simulink model "PenduloCarro"  (R2017b)
settings: Solver=ode4  StartTime=0.0  StopTime=10  FixedStep=0.0001  RelTol=1e-3
values from neighbouring files (symbols this model uses):
  g = 9.81    [PenduloInvertido.m]
  l = 0.5    [PenduloInvertido.m]
  m = 0.1    [PenduloInvertido.m]
  M = 2    [PenduloInvertido.m]
settings Model: Creator=Benjamin Nicolas  LastModifiedBy=Benjamin Nicolas

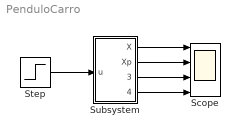
== system PenduloCarro ==
  Scope : Scope  NumInputPorts=4
  Step : Step  Time=0  SampleTime=0
  Subsystem : Subsystem
  wires:
  Subsystem/1(X) -> Scope/1
  Subsystem/2(Xp) -> Scope/2
  Subsystem/3(Theta) -> Scope/3
  Subsystem/4(Thetap) -> Scope/4
  Step/1 -> Subsystem/1("u ")

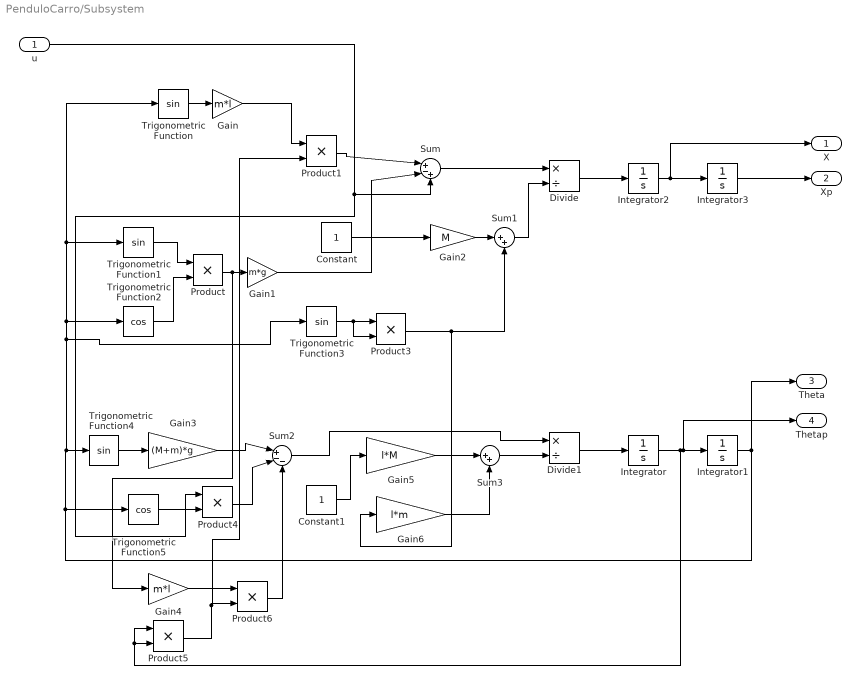
== system PenduloCarro/Subsystem ==
  "u " : Inport
  Constant : Constant
  Constant1 : Constant
  Divide : Product  Inputs=*/
  Divide1 : Product  Inputs=*/
  Gain : Gain  Gain=m*l
  Gain1 : Gain  Gain=m*g
  Gain2 : Gain  Gain=M
  Gain3 : Gain  Gain=(M+m)*g
  Gain4 : Gain  Gain=m*l
  Gain5 : Gain  Gain=l*M
  Gain6 : Gain  Gain=l*m
  Integrator{,1..3} (4 alike) : Integrator
  Product{,1,3..6} (6 alike) : Product
  Sum : Sum  Inputs=|+-+
  Sum1 : Sum  Inputs=|++
  Sum2 : Sum  Inputs=|+--
  Sum3 : Sum  Inputs=|++
  Trigonometric Function{,1,3..4} (4 alike) : Trigonometry
  Trigonometric Function2 : Trigonometry  Operator=cos
  Trigonometric Function5 : Trigonometry  Operator=cos
  X : Outport
  Xp : Outport  Port=2
  Theta : Outport  Port=3
  Thetap : Outport  Port=4
  wires:
  Gain3/1 -> Sum2/1
  Gain4/1 -> Product6/1
  Product3/1 -> Gain6/1, Sum1/2
  Gain1/1 -> Sum/2
  Trigonometric Function3/1 -> Product3/2, Product3/1
  Sum1/1 -> Divide/2
  Gain2/1 -> Sum1/1
  Product5/1 -> Product1/2, Product6/2
  Product6/1 -> Sum2/3
  Sum/1 -> Divide/1
  Product/1 -> Gain4/1, Gain1/1
  Trigonometric Function1/1 -> Product/1
  Gain6/1 -> Sum3/2
  Constant1/1 -> Gain5/1
  Trigonometric Function2/1 -> Product/2
  Trigonometric Function/1 -> Gain/1
  Integrator/1 -> Product5/2, Product5/1, Thetap/1, Integrator1/1
  Constant/1 -> Gain2/1
  Gain/1 -> Product1/1
  "u "/1 -> Product4/1, Sum/3
  Integrator2/1 -> X/1, Integrator3/1
  Integrator3/1 -> Xp/1
  Product4/1 -> Sum2/2
  Integrator1/1 -> Trigonometric Function5/1, Trigonometric Function3/1, Trigonometric Function2/1, Trigonometric Function1/1, Trigonometric Function/1, Trigonometric Function4/1, Theta/1
  Sum2/1 -> Divide1/1
  Trigonometric Function5/1 -> Product4/2
  Sum3/1 -> Divide1/2
  Trigonometric Function4/1 -> Gain3/1
  Divide/1 -> Integrator2/1
  Gain5/1 -> Sum3/1
  Divide1/1 -> Integrator/1
  Product1/1 -> Sum/1
